simulink model "edge_call_outputEvent_mulBrodcast_eg_rising"  (R2018a)
settings: Solver=FixedStepAuto  StartTime=0.0  StopTime=10.0  FixedStep=1  MaxStep=1  RelTol=1e-3
settings Model: Creator=86188  LastModifiedBy=86188

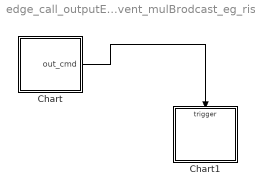
== system edge_call_outputEvent_mulBrodcast_eg_rising ==
  Chart : Stateflow chart  TreatAsAtomicUnit=on
  Chart1 : Stateflow chart  TreatAsAtomicUnit=on
  wires:
  Chart/1(out_cmd) -> Chart1/Trigger

== stateflow chart edge_call_outputEvent_mulBrodcast_eg_rising/Chart1 ==
  state AA
    en:f("en_AA");
    du:f("du_AA");
  (default) -> AA : {y = y + 1;}
  data: s function_input; y local =0
  events: out_cmd input RISING_EDGE_EVENT
  function f(s):
    | function f(s)
    |   fprintf(s+"\n");

== stateflow chart edge_call_outputEvent_mulBrodcast_eg_rising/Chart ==
  state ENTRY
    en:f("en_ENTRY");
  state A
    en:
    f("en_A");
    send(out_cmd);
    send(out_cmd);
    send(out_cmd);
    send(out_cmd);
  state B
  (default) -> ENTRY
  A -> B
  ENTRY -> A
  data: s function_input
  events: out_cmd output EITHER_EDGE_EVENT
  function f(s):
    | function f(s)
    |   fprintf(s+"\n");
